simulink model "receiver_overall_reset"  (Simulink 7.5)
settings: Solver=FixedStepDiscrete  SolverMode=SingleTasking  StartTime=0.0  StopTime=(length(simin.signals.values)-1)/Fs  FixedStep=1  RelTol=1e-3
undefined symbols (not defined in the file): Fs
libraries: xbsIndex_r4 x962
(part 4 of 9)

== system receiver_overall_reset/Receiver/Sym-Chooser/6-14/Corr0 ==
  In1 : Inport
  AddSub : xbsIndex_r4/AddSub  mode=Subtraction  use_carryin=off  use_carryout=off  en=off  latency=0  precision=Full  arith_type=Unsigned  n_bits=16  bin_pt=14  quantization=Truncate  overflow=Wrap  dbl_ovrd=off  use_behavioral_HDL=off  hw_selection=Fabric  pipelined=off  block_type=addsub
      settings: xl_area=[4 0 0 6 0 0 0]  block_version=12.1
  Constant0 : xbsIndex_r4/Constant  arith_type=Unsigned  const=chip_a  n_bits=31  bin_pt=0  explicit_period=off  period=1/8  equ=P=C  opselect=C  inp2=PCIN>>17  opr=+  inp1=P  carry=CIN  dbl_ovrd=off  block_type=constant
      settings: block_version=12.1
  Constant1 : xbsIndex_r4/Constant  arith_type=Unsigned  const=31  n_bits=5  bin_pt=0  explicit_period=off  period=1/8  equ=P=C  opselect=C  inp2=PCIN>>17  opr=+  inp1=P  carry=CIN  dbl_ovrd=off  block_type=constant
      settings: block_version=12.1
  Corr : Subsystem
  Delay_Line : Subsystem  mask{bits=31}
      mask prompts: bits "Number of Bits [2-40]"
      mask init: same as receiver_overall_reset/Receiver/Sym-Clk/Corr/Delay_Line
      mask StyleString: popup(2|3|4|5|6|7|8|9|10|11|12|13|14|15|16|17|18|19|20|21|22|23|24|25|26|27|28|29|30|31|32|33|34|35|36|37|38|39|40)
  Logical : xbsIndex_r4/Logical  logical_function=XNOR  inputs=2  en=off  latency=0  precision=User Defined  arith_type=Unsigned  n_bits=32  bin_pt=0  align_bp=on  dbl_ovrd=off  block_type=logical
      settings: xl_area=[31 0 0 31 0 0 0]  block_version=12.1
  Shift : xbsIndex_r4/Shift  shift_dir=Left  shift_bits=1  en=off  latency=0  precision=Full  arith_type=Unsigned  n_bits=7  bin_pt=0  quantization=Truncate  overflow=Wrap  dbl_ovrd=off  block_type=shift
      settings: xl_area=[0 0 0 0 0 0 0]  block_version=12.1
  Out1 : Outport
  wires:
  Constant0/1 -> Logical/2
  Delay_Line/1(Out2) -> Logical/1
  Logical/1 -> Corr/1(In1)
  Constant1/1 -> AddSub/2
  Corr/1(Out2) -> Shift/1
  Shift/1 -> AddSub/1
  In1/1 -> Delay_Line/1(In1)
  AddSub/1 -> Out1/1

== system receiver_overall_reset/Receiver/Sym-Chooser/7-15/Corr0 ==
  In1 : Inport
  AddSub : xbsIndex_r4/AddSub  mode=Subtraction  use_carryin=off  use_carryout=off  en=off  latency=0  precision=Full  arith_type=Unsigned  n_bits=16  bin_pt=14  quantization=Truncate  overflow=Wrap  dbl_ovrd=off  use_behavioral_HDL=off  hw_selection=Fabric  pipelined=off  block_type=addsub
      settings: xl_area=[4 0 0 6 0 0 0]  block_version=12.1
  Constant0 : xbsIndex_r4/Constant  arith_type=Unsigned  const=chip_a  n_bits=31  bin_pt=0  explicit_period=off  period=1/8  equ=P=C  opselect=C  inp2=PCIN>>17  opr=+  inp1=P  carry=CIN  dbl_ovrd=off  block_type=constant
      settings: block_version=12.1
  Constant1 : xbsIndex_r4/Constant  arith_type=Unsigned  const=31  n_bits=5  bin_pt=0  explicit_period=off  period=1/8  equ=P=C  opselect=C  inp2=PCIN>>17  opr=+  inp1=P  carry=CIN  dbl_ovrd=off  block_type=constant
      settings: block_version=12.1
  Corr : Subsystem
  Delay_Line : Subsystem  mask{bits=31}
      mask prompts: bits "Number of Bits [2-40]"
      mask init: same as receiver_overall_reset/Receiver/Sym-Clk/Corr/Delay_Line
      mask StyleString: popup(2|3|4|5|6|7|8|9|10|11|12|13|14|15|16|17|18|19|20|21|22|23|24|25|26|27|28|29|30|31|32|33|34|35|36|37|38|39|40)
  Logical : xbsIndex_r4/Logical  logical_function=XNOR  inputs=2  en=off  latency=0  precision=User Defined  arith_type=Unsigned  n_bits=32  bin_pt=0  align_bp=on  dbl_ovrd=off  block_type=logical
      settings: xl_area=[31 0 0 31 0 0 0]  block_version=12.1
  Shift : xbsIndex_r4/Shift  shift_dir=Left  shift_bits=1  en=off  latency=0  precision=Full  arith_type=Unsigned  n_bits=7  bin_pt=0  quantization=Truncate  overflow=Wrap  dbl_ovrd=off  block_type=shift
      settings: xl_area=[0 0 0 0 0 0 0]  block_version=12.1
  Out1 : Outport
  wires:
  Constant0/1 -> Logical/2
  Delay_Line/1(Out2) -> Logical/1
  Logical/1 -> Corr/1(In1)
  Constant1/1 -> AddSub/2
  Corr/1(Out2) -> Shift/1
  Shift/1 -> AddSub/1
  In1/1 -> Delay_Line/1(In1)
  AddSub/1 -> Out1/1

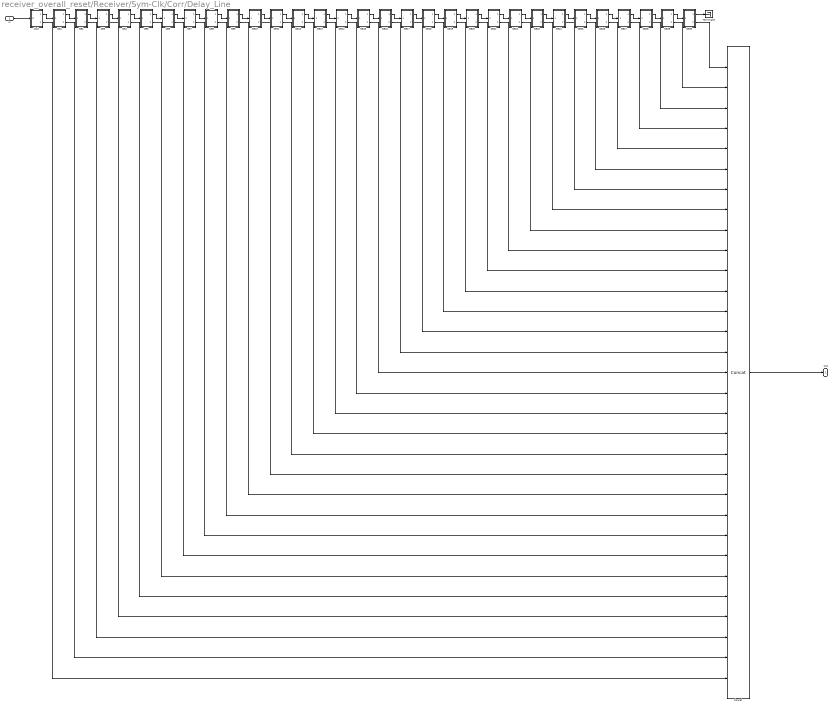
== system receiver_overall_reset/Receiver/Sym-Clk/Corr/Delay_Line ==
  In : Inport
  1to2 : Subsystem
  Concat : xbsIndex_r4/Concat  num_inputs=31  dbl_ovrd=off  block_type=concat
      settings: block_version=12.1
  DE1 : Subsystem
      mask Display: disp('z^{-1}','texmode','on')
  DE10 : Subsystem
      mask Display: disp('z^{-1}','texmode','on')
  DE11 : Subsystem
      mask Display: disp('z^{-1}','texmode','on')
  DE12 : Subsystem
      mask Display: disp('z^{-1}','texmode','on')
  DE13 : Subsystem
      mask Display: disp('z^{-1}','texmode','on')
  DE14 : Subsystem
      mask Display: disp('z^{-1}','texmode','on')
  DE15 : Subsystem
      mask Display: disp('z^{-1}','texmode','on')
  DE16 : Subsystem
      mask Display: disp('z^{-1}','texmode','on')
  DE17 : Subsystem
      mask Display: disp('z^{-1}','texmode','on')
  DE18 : Subsystem
      mask Display: disp('z^{-1}','texmode','on')
  DE19 : Subsystem
      mask Display: disp('z^{-1}','texmode','on')
  DE2 : Subsystem
      mask Display: disp('z^{-1}','texmode','on')
  DE20 : Subsystem
      mask Display: disp('z^{-1}','texmode','on')
  DE21 : Subsystem
      mask Display: disp('z^{-1}','texmode','on')
  DE22 : Subsystem
      mask Display: disp('z^{-1}','texmode','on')
  DE23 : Subsystem
      mask Display: disp('z^{-1}','texmode','on')
  DE24 : Subsystem
      mask Display: disp('z^{-1}','texmode','on')
  DE25 : Subsystem
      mask Display: disp('z^{-1}','texmode','on')
  DE26 : Subsystem
      mask Display: disp('z^{-1}','texmode','on')
  DE27 : Subsystem
      mask Display: disp('z^{-1}','texmode','on')
  DE28 : Subsystem
      mask Display: disp('z^{-1}','texmode','on')
  DE29 : Subsystem
      mask Display: disp('z^{-1}','texmode','on')
  DE3 : Subsystem
      mask Display: disp('z^{-1}','texmode','on')
  DE30 : Subsystem
      mask Display: disp('z^{-1}','texmode','on')
  DE4 : Subsystem
      mask Display: disp('z^{-1}','texmode','on')
  DE5 : Subsystem
      mask Display: disp('z^{-1}','texmode','on')
  DE6 : Subsystem
      mask Display: disp('z^{-1}','texmode','on')
  DE7 : Subsystem
      mask Display: disp('z^{-1}','texmode','on')
  DE8 : Subsystem
      mask Display: disp('z^{-1}','texmode','on')
  DE9 : Subsystem
      mask Display: disp('z^{-1}','texmode','on')
  Terminator : Terminator
  Out : Outport
  wires:
  Concat/1 -> Out/1
  In/1 -> 1to2/1(In)
  1to2/1(Out1) -> DE1/1(In1)
  DE30/1(Out1) -> Terminator/1
  1to2/2(Out2) -> Concat/31
  DE1/2(Out2) -> Concat/30
  DE2/2(Out2) -> Concat/29
  DE3/2(Out2) -> Concat/28
  DE4/2(Out2) -> Concat/27
  DE5/2(Out2) -> Concat/26
  DE6/2(Out2) -> Concat/25
  DE7/2(Out2) -> Concat/24
  DE8/2(Out2) -> Concat/23
  DE9/2(Out2) -> Concat/22
  DE10/2(Out2) -> Concat/21
  DE11/2(Out2) -> Concat/20
  DE12/2(Out2) -> Concat/19
  DE13/2(Out2) -> Concat/18
  DE14/2(Out2) -> Concat/17
  DE15/2(Out2) -> Concat/16
  DE16/2(Out2) -> Concat/15
  DE17/2(Out2) -> Concat/14
  DE18/2(Out2) -> Concat/13
  DE19/2(Out2) -> Concat/12
  DE20/2(Out2) -> Concat/11
  DE21/2(Out2) -> Concat/10
  DE22/2(Out2) -> Concat/9
  DE23/2(Out2) -> Concat/8
  DE24/2(Out2) -> Concat/7
  DE25/2(Out2) -> Concat/6
  DE26/2(Out2) -> Concat/5
  DE27/2(Out2) -> Concat/4
  DE28/2(Out2) -> Concat/3
  DE29/2(Out2) -> Concat/2
  DE30/2(Out2) -> Concat/1
  DE2/1(Out1) -> DE3/1(In1)
  DE3/1(Out1) -> DE4/1(In1)
  DE4/1(Out1) -> DE5/1(In1)
  DE5/1(Out1) -> DE6/1(In1)
  DE6/1(Out1) -> DE7/1(In1)
  DE7/1(Out1) -> DE8/1(In1)
  DE8/1(Out1) -> DE9/1(In1)
  DE9/1(Out1) -> DE10/1(In1)
  DE10/1(Out1) -> DE11/1(In1)
  DE11/1(Out1) -> DE12/1(In1)
  DE12/1(Out1) -> DE13/1(In1)
  DE13/1(Out1) -> DE14/1(In1)
  DE14/1(Out1) -> DE15/1(In1)
  DE15/1(Out1) -> DE16/1(In1)
  DE16/1(Out1) -> DE17/1(In1)
  DE17/1(Out1) -> DE18/1(In1)
  DE18/1(Out1) -> DE19/1(In1)
  DE19/1(Out1) -> DE20/1(In1)
  DE20/1(Out1) -> DE21/1(In1)
  DE21/1(Out1) -> DE22/1(In1)
  DE22/1(Out1) -> DE23/1(In1)
  DE23/1(Out1) -> DE24/1(In1)
  DE24/1(Out1) -> DE25/1(In1)
  DE25/1(Out1) -> DE26/1(In1)
  DE26/1(Out1) -> DE27/1(In1)
  DE27/1(Out1) -> DE28/1(In1)
  DE28/1(Out1) -> DE29/1(In1)
  DE29/1(Out1) -> DE30/1(In1)
  DE1/1(Out1) -> DE2/1(In1)

== system receiver_overall_reset/Receiver/Sym-Clk/Corr/count 1s ==
  in : Inport
  0-3 : xbsIndex_r4/Slice  nbits=4  boolean_output=off  mode=Lower Bit Location + Width  bit1=0  base1=MSB of Input  bit0=0  base0=LSB of Input  dbl_ovrd=off  block_type=slice
      settings: block_version=12.1
  12-15 : xbsIndex_r4/Slice  nbits=4  boolean_output=off  mode=Lower Bit Location + Width  bit1=-12  base1=MSB of Input  bit0=12  base0=LSB of Input  dbl_ovrd=off  block_type=slice
      settings: block_version=12.1
  16-19 : xbsIndex_r4/Slice  nbits=4  boolean_output=off  mode=Lower Bit Location + Width  bit1=0  base1=LSB of Input  bit0=16  base0=LSB of Input  dbl_ovrd=off  block_type=slice
      settings: block_version=12.1
  20-23 : xbsIndex_r4/Slice  nbits=4  boolean_output=off  mode=Lower Bit Location + Width  bit1=0  base1=LSB of Input  bit0=20  base0=LSB of Input  dbl_ovrd=off  block_type=slice
      settings: block_version=12.1
  24-27 : xbsIndex_r4/Slice  nbits=4  boolean_output=off  mode=Lower Bit Location + Width  bit1=0  base1=LSB of Input  bit0=24  base0=LSB of Input  dbl_ovrd=off  block_type=slice
      settings: block_version=12.1
  28-31 : xbsIndex_r4/Slice  nbits=4  boolean_output=off  mode=Lower Bit Location + Width  bit1=0  base1=LSB of Input  bit0=28  base0=LSB of Input  dbl_ovrd=off  block_type=slice
      settings: block_version=12.1
  4-7 : xbsIndex_r4/Slice  nbits=4  boolean_output=off  mode=Lower Bit Location + Width  bit1=-4  base1=MSB of Input  bit0=4  base0=LSB of Input  dbl_ovrd=off  block_type=slice
      settings: block_version=12.1
  8-11 : xbsIndex_r4/Slice  nbits=4  boolean_output=off  mode=Lower Bit Location + Width  bit1=-8  base1=MSB of Input  bit0=8  base0=LSB of Input  dbl_ovrd=off  block_type=slice
      settings: block_version=12.1
  AddSub2 : xbsIndex_r4/AddSub  mode=Addition  use_carryin=off  use_carryout=off  en=off  latency=0  precision=Full  arith_type=Unsigned  n_bits=16  bin_pt=14  quantization=Truncate  overflow=Wrap  dbl_ovrd=off  use_behavioral_HDL=off  hw_selection=Fabric  pipelined=off  block_type=addsub
      settings: xl_area=[3 0 0 4 0 0 0]  block_version=12.1
  AddSub3 : xbsIndex_r4/AddSub  mode=Addition  use_carryin=off  use_carryout=off  en=off  latency=0  precision=Full  arith_type=Unsigned  n_bits=16  bin_pt=14  quantization=Truncate  overflow=Wrap  dbl_ovrd=off  use_behavioral_HDL=off  hw_selection=Fabric  pipelined=off  block_type=addsub
      settings: xl_area=[3 0 0 5 0 0 0]  block_version=12.1
  AddSub6 : xbsIndex_r4/AddSub  mode=Addition  use_carryin=off  use_carryout=off  en=off  latency=0  precision=Full  arith_type=Unsigned  n_bits=16  bin_pt=14  quantization=Truncate  overflow=Wrap  dbl_ovrd=off  use_behavioral_HDL=off  hw_selection=Fabric  pipelined=off  block_type=addsub
      settings: xl_area=[3 0 0 4 0 0 0]  block_version=12.1
  LUT{0..7} (8 alike) : xbsIndex_r4/ROM  depth=16  initVector=[0,1,1,2,1,2,2,3,1,2,2,3,2,3,3,4]  distributed_mem=Distributed memory  rst=off  init_reg=0  en=off  latency=0  arith_type=Unsigned  n_bits=3  bin_pt=0  dbl_ovrd=off  optimize=Area  use_rpm=on  block_type=sprom
      settings: xl_area=[0 0 1 0 0 0 0]  block_version=12.1
  add{1..4} (4 alike) : xbsIndex_r4/AddSub  mode=Addition  use_carryin=off  use_carryout=off  en=off  latency=0  precision=Full  arith_type=Unsigned  n_bits=16  bin_pt=14  quantization=Truncate  overflow=Wrap  dbl_ovrd=off  use_behavioral_HDL=off  hw_selection=Fabric  pipelined=off  block_type=addsub
      settings: xl_area=[2 0 0 3 0 0 0]  block_version=12.1
  out : Outport
  wires:
  in/1 -> 0-3/1, 12-15/1, 28-31/1, 24-27/1, 20-23/1, 16-19/1, 8-11/1, 4-7/1
  0-3/1 -> LUT0/1
  12-15/1 -> LUT3/1
  8-11/1 -> LUT2/1
  4-7/1 -> LUT1/1
  LUT0/1 -> add1/1
  LUT1/1 -> add1/2
  LUT2/1 -> add2/1
  LUT3/1 -> add2/2
  add2/1 -> AddSub2/2
  add1/1 -> AddSub2/1
  AddSub3/1 -> out/1
  16-19/1 -> LUT4/1
  28-31/1 -> LUT7/1
  24-27/1 -> LUT6/1
  20-23/1 -> LUT5/1
  LUT4/1 -> add3/1
  LUT5/1 -> add3/2
  LUT6/1 -> add4/1
  LUT7/1 -> add4/2
  add4/1 -> AddSub6/2
  add3/1 -> AddSub6/1
  AddSub2/1 -> AddSub3/1
  AddSub6/1 -> AddSub3/2

== system receiver_overall_reset/Receiver/FM demod/CORDIC ATAN/CORDIC Fine Angle PE/CORDIC PE1 ==
  note: X = x - y if y < 0, otherwise
      |    = x + y
      | Y = y + x if y < 0, otherwise
      |    = y - x
      | Z = z - atan(1/2^i) if y < 0, otherwise
      |    = z + atan(1/2^i)
  x : Inport  OutDataType=sfix(16)  OutScaling=2^0
  y : Inport  Port=2  OutDataType=sfix(16)  OutScaling=2^0
  z : Inport  Port=3  OutDataType=sfix(16)  OutScaling=2^0
  AddSub : xbsIndex_r4/AddSub  mode=Addition or Subtraction  use_carryin=off  use_carryout=off  en=off  latency=pipeline  precision=User Defined  arith_type="Signed  (2's comp)"  n_bits=pe_nbits  bin_pt=pe_binpt  quantization=Truncate  overflow=Wrap  dbl_ovrd=off  use_behavioral_HDL=on  hw_selection=Fabric  pipelined=off  use_rpm=off  block_type=addsub
      settings: xl_area=[17 0 0 33 0 0 0]  block_version=VER_STRING_GOES_HERE
  AddSub1 : xbsIndex_r4/AddSub  mode=Addition or Subtraction  use_carryin=off  use_carryout=off  en=off  latency=pipeline  precision=User Defined  arith_type="Signed  (2's comp)"  n_bits=pe_nbits  bin_pt=pe_binpt  quantization=Truncate  overflow=Wrap  dbl_ovrd=off  use_behavioral_HDL=on  hw_selection=Fabric  pipelined=off  use_rpm=off  block_type=addsub
      settings: xl_area=[17 0 0 33 0 0 0]  block_version=VER_STRING_GOES_HERE
  AddSub2 : xbsIndex_r4/AddSub  mode=Addition or Subtraction  use_carryin=off  use_carryout=off  en=off  latency=pipeline  precision=User Defined  arith_type="Signed  (2's comp)"  n_bits=pe_nbits  bin_pt=pe_binpt  quantization=Truncate  overflow=Wrap  dbl_ovrd=off  use_behavioral_HDL=on  hw_selection=Fabric  pipelined=off  use_rpm=off  block_type=addsub
      settings: xl_area=[17 0 0 33 0 0 0]  block_version=VER_STRING_GOES_HERE
  Constant : xbsIndex_r4/Constant  arith_type=Signed (2's comp)  const=epsilon_k  n_bits=pe_nbits  bin_pt=pe_binpt  explicit_period=off  period=1  equ=P=C  opselect=C  inp2=PCIN>>17  opr=+  inp1=P  carry=CIN  dbl_ovrd=off  block_type=constant
      settings: block_version=VER_STRING_GOES_HERE
  Inverter : xbsIndex_r4/Inverter  en=off  latency=0  dbl_ovrd=off  block_type=inv
      settings: xl_area=[0 0 0 0 0 0 0]  block_version=VER_STRING_GOES_HERE
  Shift : xbsIndex_r4/Shift  shift_dir=Right  shift_bits=ii  en=off  latency=0  precision=User Defined  arith_type="Signed  (2's comp)"  n_bits=pe_nbits  bin_pt=pe_binpt  quantization=Truncate  overflow=Wrap  dbl_ovrd=off  block_type=shift
      settings: xl_area=[0 0 0 0 0 0 0]  block_version=VER_STRING_GOES_HERE
  Shift1 : xbsIndex_r4/Shift  shift_dir=Right  shift_bits=ii  en=off  latency=0  precision=User Defined  arith_type="Signed  (2's comp)"  n_bits=pe_nbits  bin_pt=pe_binpt  quantization=Truncate  overflow=Wrap  dbl_ovrd=off  block_type=shift
      settings: xl_area=[0 0 0 0 0 0 0]  block_version=VER_STRING_GOES_HERE
  Slice : xbsIndex_r4/Slice  nbits=1  boolean_output=on  mode=Upper Bit Location + Width  bit1=0  base1=MSB of Input  bit0=0  base0=LSB of Input  dbl_ovrd=off  block_type=slice
      settings: infoedit="Extracts a given range of bits from each input sample and presents it at the output.  The output type is ordinarily unsigned with binary point at zero, but can be Boolean when the slice is one bit wide.<P><P>Hardware notes: In hardware this block costs nothing."  block_version=VER_STRING_GOES_HERE
  X : Outport  OutDataType=sfix(16)  OutScaling=2^0
  Y : Outport  Port=2  OutDataType=sfix(16)  OutScaling=2^0
  Z : Outport  Port=3  OutDataType=sfix(16)  OutScaling=2^0
  wires:
  Slice/1 -> AddSub/3, AddSub2/3, Inverter/1
  Shift1/1 -> AddSub/2
  Shift/1 -> AddSub1/2
  Inverter/1 -> AddSub1/3
  Constant/1 -> AddSub2/2
  AddSub2/1 -> Z/1
  AddSub1/1 -> Y/1
  z/1 -> AddSub2/1
  AddSub/1 -> X/1
  y/1 -> Slice/1, Shift1/1, AddSub1/1
  x/1 -> Shift/1, AddSub/1

== system receiver_overall_reset/Receiver/FM demod/CORDIC ATAN/CORDIC Fine Angle PE/CORDIC PE2 ==
  note: X = x - y if y < 0, otherwise
      |    = x + y
      | Y = y + x if y < 0, otherwise
      |    = y - x
      | Z = z - atan(1/2^i) if y < 0, otherwise
      |    = z + atan(1/2^i)
  x : Inport  OutDataType=sfix(16)  OutScaling=2^0
  y : Inport  Port=2  OutDataType=sfix(16)  OutScaling=2^0
  z : Inport  Port=3  OutDataType=sfix(16)  OutScaling=2^0
  AddSub : xbsIndex_r4/AddSub  mode=Addition or Subtraction  use_carryin=off  use_carryout=off  en=off  latency=pipeline  precision=User Defined  arith_type="Signed  (2's comp)"  n_bits=pe_nbits  bin_pt=pe_binpt  quantization=Truncate  overflow=Wrap  dbl_ovrd=off  use_behavioral_HDL=on  hw_selection=Fabric  pipelined=off  use_rpm=off  block_type=addsub
      settings: xl_area=[17 0 0 33 0 0 0]  block_version=VER_STRING_GOES_HERE
  AddSub1 : xbsIndex_r4/AddSub  mode=Addition or Subtraction  use_carryin=off  use_carryout=off  en=off  latency=pipeline  precision=User Defined  arith_type="Signed  (2's comp)"  n_bits=pe_nbits  bin_pt=pe_binpt  quantization=Truncate  overflow=Wrap  dbl_ovrd=off  use_behavioral_HDL=on  hw_selection=Fabric  pipelined=off  use_rpm=off  block_type=addsub
      settings: xl_area=[17 0 0 33 0 0 0]  block_version=VER_STRING_GOES_HERE
  AddSub2 : xbsIndex_r4/AddSub  mode=Addition or Subtraction  use_carryin=off  use_carryout=off  en=off  latency=pipeline  precision=User Defined  arith_type="Signed  (2's comp)"  n_bits=pe_nbits  bin_pt=pe_binpt  quantization=Truncate  overflow=Wrap  dbl_ovrd=off  use_behavioral_HDL=on  hw_selection=Fabric  pipelined=off  use_rpm=off  block_type=addsub
      settings: xl_area=[17 0 0 33 0 0 0]  block_version=VER_STRING_GOES_HERE
  Constant : xbsIndex_r4/Constant  arith_type=Signed (2's comp)  const=epsilon_k  n_bits=pe_nbits  bin_pt=pe_binpt  explicit_period=off  period=1  equ=P=C  opselect=C  inp2=PCIN>>17  opr=+  inp1=P  carry=CIN  dbl_ovrd=off  block_type=constant
      settings: block_version=VER_STRING_GOES_HERE
  Inverter : xbsIndex_r4/Inverter  en=off  latency=0  dbl_ovrd=off  block_type=inv
      settings: xl_area=[0 0 0 0 0 0 0]  block_version=VER_STRING_GOES_HERE
  Shift : xbsIndex_r4/Shift  shift_dir=Right  shift_bits=ii  en=off  latency=0  precision=User Defined  arith_type="Signed  (2's comp)"  n_bits=pe_nbits  bin_pt=pe_binpt  quantization=Truncate  overflow=Wrap  dbl_ovrd=off  block_type=shift
      settings: xl_area=[0 0 0 0 0 0 0]  block_version=VER_STRING_GOES_HERE
  Shift1 : xbsIndex_r4/Shift  shift_dir=Right  shift_bits=ii  en=off  latency=0  precision=User Defined  arith_type="Signed  (2's comp)"  n_bits=pe_nbits  bin_pt=pe_binpt  quantization=Truncate  overflow=Wrap  dbl_ovrd=off  block_type=shift
      settings: xl_area=[0 0 0 0 0 0 0]  block_version=VER_STRING_GOES_HERE
  Slice : xbsIndex_r4/Slice  nbits=1  boolean_output=on  mode=Upper Bit Location + Width  bit1=0  base1=MSB of Input  bit0=0  base0=LSB of Input  dbl_ovrd=off  block_type=slice
      settings: infoedit="Extracts a given range of bits from each input sample and presents it at the output.  The output type is ordinarily unsigned with binary point at zero, but can be Boolean when the slice is one bit wide.<P><P>Hardware notes: In hardware this block costs nothing."  block_version=VER_STRING_GOES_HERE
  X : Outport  OutDataType=sfix(16)  OutScaling=2^0
  Y : Outport  Port=2  OutDataType=sfix(16)  OutScaling=2^0
  Z : Outport  Port=3  OutDataType=sfix(16)  OutScaling=2^0
  wires:
  x/1 -> AddSub/1, Shift/1
  y/1 -> AddSub1/1, Shift1/1, Slice/1
  AddSub/1 -> X/1
  z/1 -> AddSub2/1
  AddSub1/1 -> Y/1
  AddSub2/1 -> Z/1
  Constant/1 -> AddSub2/2
  Inverter/1 -> AddSub1/3
  Shift/1 -> AddSub1/2
  Shift1/1 -> AddSub/2
  Slice/1 -> Inverter/1, AddSub2/3, AddSub/3

== system receiver_overall_reset/Receiver/FM demod/CORDIC ATAN/CORDIC Fine Angle PE/CORDIC PE3 ==
  note: X = x - y if y < 0, otherwise
      |    = x + y
      | Y = y + x if y < 0, otherwise
      |    = y - x
      | Z = z - atan(1/2^i) if y < 0, otherwise
      |    = z + atan(1/2^i)
  x : Inport  OutDataType=sfix(16)  OutScaling=2^0
  y : Inport  Port=2  OutDataType=sfix(16)  OutScaling=2^0
  z : Inport  Port=3  OutDataType=sfix(16)  OutScaling=2^0
  AddSub : xbsIndex_r4/AddSub  mode=Addition or Subtraction  use_carryin=off  use_carryout=off  en=off  latency=pipeline  precision=User Defined  arith_type="Signed  (2's comp)"  n_bits=pe_nbits  bin_pt=pe_binpt  quantization=Truncate  overflow=Wrap  dbl_ovrd=off  use_behavioral_HDL=on  hw_selection=Fabric  pipelined=off  use_rpm=off  block_type=addsub
      settings: xl_area=[17 0 0 33 0 0 0]  block_version=VER_STRING_GOES_HERE
  AddSub1 : xbsIndex_r4/AddSub  mode=Addition or Subtraction  use_carryin=off  use_carryout=off  en=off  latency=pipeline  precision=User Defined  arith_type="Signed  (2's comp)"  n_bits=pe_nbits  bin_pt=pe_binpt  quantization=Truncate  overflow=Wrap  dbl_ovrd=off  use_behavioral_HDL=on  hw_selection=Fabric  pipelined=off  use_rpm=off  block_type=addsub
      settings: xl_area=[17 0 0 33 0 0 0]  block_version=VER_STRING_GOES_HERE
  AddSub2 : xbsIndex_r4/AddSub  mode=Addition or Subtraction  use_carryin=off  use_carryout=off  en=off  latency=pipeline  precision=User Defined  arith_type="Signed  (2's comp)"  n_bits=pe_nbits  bin_pt=pe_binpt  quantization=Truncate  overflow=Wrap  dbl_ovrd=off  use_behavioral_HDL=on  hw_selection=Fabric  pipelined=off  use_rpm=off  block_type=addsub
      settings: xl_area=[17 0 0 33 0 0 0]  block_version=VER_STRING_GOES_HERE
  Constant : xbsIndex_r4/Constant  arith_type=Signed (2's comp)  const=epsilon_k  n_bits=pe_nbits  bin_pt=pe_binpt  explicit_period=off  period=1  equ=P=C  opselect=C  inp2=PCIN>>17  opr=+  inp1=P  carry=CIN  dbl_ovrd=off  block_type=constant
      settings: block_version=VER_STRING_GOES_HERE
  Inverter : xbsIndex_r4/Inverter  en=off  latency=0  dbl_ovrd=off  block_type=inv
      settings: xl_area=[0 0 0 0 0 0 0]  block_version=VER_STRING_GOES_HERE
  Shift : xbsIndex_r4/Shift  shift_dir=Right  shift_bits=ii  en=off  latency=0  precision=User Defined  arith_type="Signed  (2's comp)"  n_bits=pe_nbits  bin_pt=pe_binpt  quantization=Truncate  overflow=Wrap  dbl_ovrd=off  block_type=shift
      settings: xl_area=[0 0 0 0 0 0 0]  block_version=VER_STRING_GOES_HERE
  Shift1 : xbsIndex_r4/Shift  shift_dir=Right  shift_bits=ii  en=off  latency=0  precision=User Defined  arith_type="Signed  (2's comp)"  n_bits=pe_nbits  bin_pt=pe_binpt  quantization=Truncate  overflow=Wrap  dbl_ovrd=off  block_type=shift
      settings: xl_area=[0 0 0 0 0 0 0]  block_version=VER_STRING_GOES_HERE
  Slice : xbsIndex_r4/Slice  nbits=1  boolean_output=on  mode=Upper Bit Location + Width  bit1=0  base1=MSB of Input  bit0=0  base0=LSB of Input  dbl_ovrd=off  block_type=slice
      settings: infoedit="Extracts a given range of bits from each input sample and presents it at the output.  The output type is ordinarily unsigned with binary point at zero, but can be Boolean when the slice is one bit wide.<P><P>Hardware notes: In hardware this block costs nothing."  block_version=VER_STRING_GOES_HERE
  X : Outport  OutDataType=sfix(16)  OutScaling=2^0
  Y : Outport  Port=2  OutDataType=sfix(16)  OutScaling=2^0
  Z : Outport  Port=3  OutDataType=sfix(16)  OutScaling=2^0
  wires:
  x/1 -> AddSub/1, Shift/1
  y/1 -> AddSub1/1, Shift1/1, Slice/1
  AddSub/1 -> X/1
  z/1 -> AddSub2/1
  AddSub1/1 -> Y/1
  AddSub2/1 -> Z/1
  Constant/1 -> AddSub2/2
  Inverter/1 -> AddSub1/3
  Shift/1 -> AddSub1/2
  Shift1/1 -> AddSub/2
  Slice/1 -> Inverter/1, AddSub2/3, AddSub/3

== system receiver_overall_reset/Receiver/FM demod/CORDIC ATAN/CORDIC Fine Angle PE/CORDIC PE4 ==
  note: X = x - y if y < 0, otherwise
      |    = x + y
      | Y = y + x if y < 0, otherwise
      |    = y - x
      | Z = z - atan(1/2^i) if y < 0, otherwise
      |    = z + atan(1/2^i)
  x : Inport  OutDataType=sfix(16)  OutScaling=2^0
  y : Inport  Port=2  OutDataType=sfix(16)  OutScaling=2^0
  z : Inport  Port=3  OutDataType=sfix(16)  OutScaling=2^0
  AddSub : xbsIndex_r4/AddSub  mode=Addition or Subtraction  use_carryin=off  use_carryout=off  en=off  latency=pipeline  precision=User Defined  arith_type="Signed  (2's comp)"  n_bits=pe_nbits  bin_pt=pe_binpt  quantization=Truncate  overflow=Wrap  dbl_ovrd=off  use_behavioral_HDL=on  hw_selection=Fabric  pipelined=off  use_rpm=off  block_type=addsub
      settings: xl_area=[17 0 0 33 0 0 0]  block_version=VER_STRING_GOES_HERE
  AddSub1 : xbsIndex_r4/AddSub  mode=Addition or Subtraction  use_carryin=off  use_carryout=off  en=off  latency=pipeline  precision=User Defined  arith_type="Signed  (2's comp)"  n_bits=pe_nbits  bin_pt=pe_binpt  quantization=Truncate  overflow=Wrap  dbl_ovrd=off  use_behavioral_HDL=on  hw_selection=Fabric  pipelined=off  use_rpm=off  block_type=addsub
      settings: xl_area=[17 0 0 33 0 0 0]  block_version=VER_STRING_GOES_HERE
  AddSub2 : xbsIndex_r4/AddSub  mode=Addition or Subtraction  use_carryin=off  use_carryout=off  en=off  latency=pipeline  precision=User Defined  arith_type="Signed  (2's comp)"  n_bits=pe_nbits  bin_pt=pe_binpt  quantization=Truncate  overflow=Wrap  dbl_ovrd=off  use_behavioral_HDL=on  hw_selection=Fabric  pipelined=off  use_rpm=off  block_type=addsub
      settings: xl_area=[17 0 0 33 0 0 0]  block_version=VER_STRING_GOES_HERE
  Constant : xbsIndex_r4/Constant  arith_type=Signed (2's comp)  const=epsilon_k  n_bits=pe_nbits  bin_pt=pe_binpt  explicit_period=off  period=1  equ=P=C  opselect=C  inp2=PCIN>>17  opr=+  inp1=P  carry=CIN  dbl_ovrd=off  block_type=constant
      settings: block_version=VER_STRING_GOES_HERE
  Inverter : xbsIndex_r4/Inverter  en=off  latency=0  dbl_ovrd=off  block_type=inv
      settings: xl_area=[0 0 0 0 0 0 0]  block_version=VER_STRING_GOES_HERE
  Shift : xbsIndex_r4/Shift  shift_dir=Right  shift_bits=ii  en=off  latency=0  precision=User Defined  arith_type="Signed  (2's comp)"  n_bits=pe_nbits  bin_pt=pe_binpt  quantization=Truncate  overflow=Wrap  dbl_ovrd=off  block_type=shift
      settings: xl_area=[0 0 0 0 0 0 0]  block_version=VER_STRING_GOES_HERE
  Shift1 : xbsIndex_r4/Shift  shift_dir=Right  shift_bits=ii  en=off  latency=0  precision=User Defined  arith_type="Signed  (2's comp)"  n_bits=pe_nbits  bin_pt=pe_binpt  quantization=Truncate  overflow=Wrap  dbl_ovrd=off  block_type=shift
      settings: xl_area=[0 0 0 0 0 0 0]  block_version=VER_STRING_GOES_HERE
  Slice : xbsIndex_r4/Slice  nbits=1  boolean_output=on  mode=Upper Bit Location + Width  bit1=0  base1=MSB of Input  bit0=0  base0=LSB of Input  dbl_ovrd=off  block_type=slice
      settings: infoedit="Extracts a given range of bits from each input sample and presents it at the output.  The output type is ordinarily unsigned with binary point at zero, but can be Boolean when the slice is one bit wide.<P><P>Hardware notes: In hardware this block costs nothing."  block_version=VER_STRING_GOES_HERE
  X : Outport  OutDataType=sfix(16)  OutScaling=2^0
  Y : Outport  Port=2  OutDataType=sfix(16)  OutScaling=2^0
  Z : Outport  Port=3  OutDataType=sfix(16)  OutScaling=2^0
  wires:
  x/1 -> AddSub/1, Shift/1
  y/1 -> AddSub1/1, Shift1/1, Slice/1
  AddSub/1 -> X/1
  z/1 -> AddSub2/1
  AddSub1/1 -> Y/1
  AddSub2/1 -> Z/1
  Constant/1 -> AddSub2/2
  Inverter/1 -> AddSub1/3
  Shift/1 -> AddSub1/2
  Shift1/1 -> AddSub/2
  Slice/1 -> Inverter/1, AddSub2/3, AddSub/3

== system receiver_overall_reset/Receiver/FM demod/CORDIC ATAN/CORDIC Fine Angle PE/CORDIC PE5 ==
  note: X = x - y if y < 0, otherwise
      |    = x + y
      | Y = y + x if y < 0, otherwise
      |    = y - x
      | Z = z - atan(1/2^i) if y < 0, otherwise
      |    = z + atan(1/2^i)
  x : Inport  OutDataType=sfix(16)  OutScaling=2^0
  y : Inport  Port=2  OutDataType=sfix(16)  OutScaling=2^0
  z : Inport  Port=3  OutDataType=sfix(16)  OutScaling=2^0
  AddSub : xbsIndex_r4/AddSub  mode=Addition or Subtraction  use_carryin=off  use_carryout=off  en=off  latency=pipeline  precision=User Defined  arith_type="Signed  (2's comp)"  n_bits=pe_nbits  bin_pt=pe_binpt  quantization=Truncate  overflow=Wrap  dbl_ovrd=off  use_behavioral_HDL=on  hw_selection=Fabric  pipelined=off  use_rpm=off  block_type=addsub
      settings: xl_area=[17 0 0 33 0 0 0]  block_version=VER_STRING_GOES_HERE
  AddSub1 : xbsIndex_r4/AddSub  mode=Addition or Subtraction  use_carryin=off  use_carryout=off  en=off  latency=pipeline  precision=User Defined  arith_type="Signed  (2's comp)"  n_bits=pe_nbits  bin_pt=pe_binpt  quantization=Truncate  overflow=Wrap  dbl_ovrd=off  use_behavioral_HDL=on  hw_selection=Fabric  pipelined=off  use_rpm=off  block_type=addsub
      settings: xl_area=[17 0 0 33 0 0 0]  block_version=VER_STRING_GOES_HERE
  AddSub2 : xbsIndex_r4/AddSub  mode=Addition or Subtraction  use_carryin=off  use_carryout=off  en=off  latency=pipeline  precision=User Defined  arith_type="Signed  (2's comp)"  n_bits=pe_nbits  bin_pt=pe_binpt  quantization=Truncate  overflow=Wrap  dbl_ovrd=off  use_behavioral_HDL=on  hw_selection=Fabric  pipelined=off  use_rpm=off  block_type=addsub
      settings: xl_area=[17 0 0 33 0 0 0]  block_version=VER_STRING_GOES_HERE
  Constant : xbsIndex_r4/Constant  arith_type=Signed (2's comp)  const=epsilon_k  n_bits=pe_nbits  bin_pt=pe_binpt  explicit_period=off  period=1  equ=P=C  opselect=C  inp2=PCIN>>17  opr=+  inp1=P  carry=CIN  dbl_ovrd=off  block_type=constant
      settings: block_version=VER_STRING_GOES_HERE
  Inverter : xbsIndex_r4/Inverter  en=off  latency=0  dbl_ovrd=off  block_type=inv
      settings: xl_area=[0 0 0 0 0 0 0]  block_version=VER_STRING_GOES_HERE
  Shift : xbsIndex_r4/Shift  shift_dir=Right  shift_bits=ii  en=off  latency=0  precision=User Defined  arith_type="Signed  (2's comp)"  n_bits=pe_nbits  bin_pt=pe_binpt  quantization=Truncate  overflow=Wrap  dbl_ovrd=off  block_type=shift
      settings: xl_area=[0 0 0 0 0 0 0]  block_version=VER_STRING_GOES_HERE
  Shift1 : xbsIndex_r4/Shift  shift_dir=Right  shift_bits=ii  en=off  latency=0  precision=User Defined  arith_type="Signed  (2's comp)"  n_bits=pe_nbits  bin_pt=pe_binpt  quantization=Truncate  overflow=Wrap  dbl_ovrd=off  block_type=shift
      settings: xl_area=[0 0 0 0 0 0 0]  block_version=VER_STRING_GOES_HERE
  Slice : xbsIndex_r4/Slice  nbits=1  boolean_output=on  mode=Upper Bit Location + Width  bit1=0  base1=MSB of Input  bit0=0  base0=LSB of Input  dbl_ovrd=off  block_type=slice
      settings: infoedit="Extracts a given range of bits from each input sample and presents it at the output.  The output type is ordinarily unsigned with binary point at zero, but can be Boolean when the slice is one bit wide.<P><P>Hardware notes: In hardware this block costs nothing."  block_version=VER_STRING_GOES_HERE
  X : Outport  OutDataType=sfix(16)  OutScaling=2^0
  Y : Outport  Port=2  OutDataType=sfix(16)  OutScaling=2^0
  Z : Outport  Port=3  OutDataType=sfix(16)  OutScaling=2^0
  wires:
  x/1 -> AddSub/1, Shift/1
  y/1 -> AddSub1/1, Shift1/1, Slice/1
  AddSub/1 -> X/1
  z/1 -> AddSub2/1
  AddSub1/1 -> Y/1
  AddSub2/1 -> Z/1
  Constant/1 -> AddSub2/2
  Inverter/1 -> AddSub1/3
  Shift/1 -> AddSub1/2
  Shift1/1 -> AddSub/2
  Slice/1 -> Inverter/1, AddSub2/3, AddSub/3

== system receiver_overall_reset/Receiver/Sym-Chooser/0-8/Corr0/Corr ==
  In1 : Inport
  AddSub{,1..6} (7 alike) : xbsIndex_r4/AddSub  mode=Addition  use_carryin=off  use_carryout=off  en=off  latency=0  precision=Full  arith_type=Unsigned  n_bits=16  bin_pt=14  quantization=Truncate  overflow=Wrap  dbl_ovrd=off  use_behavioral_HDL=off  hw_selection=Fabric  pipelined=off  block_type=addsub
      AddSub settings: xl_area=[2 0 0 3 0 0 0]  block_version=12.1
      AddSub1 settings: xl_area=[2 0 0 3 0 0 0]  block_version=12.1
      AddSub2 settings: xl_area=[3 0 0 4 0 0 0]  block_version=12.1
      AddSub3 settings: xl_area=[3 0 0 5 0 0 0]  block_version=12.1
      AddSub4 settings: xl_area=[2 0 0 3 0 0 0]  block_version=12.1
      AddSub5 settings: xl_area=[2 0 0 3 0 0 0]  block_version=12.1
      AddSub6 settings: xl_area=[3 0 0 4 0 0 0]  block_version=12.1
  LUT{0..7} (8 alike) : xbsIndex_r4/ROM  depth=16  initVector=[0,1,1,2,1,2,2,3,1,2,2,3,2,3,3,4]  distributed_mem=Distributed memory  rst=off  init_reg=0  en=off  latency=0  arith_type=Unsigned  n_bits=3  bin_pt=0  dbl_ovrd=off  optimize=Area  use_rpm=on  block_type=sprom
      settings: xl_area=[0 0 1 0 0 0 0]  block_version=12.1
  Slice0 : xbsIndex_r4/Slice  nbits=4  boolean_output=off  mode=Lower Bit Location + Width  bit1=0  base1=MSB of Input  bit0=0  base0=LSB of Input  dbl_ovrd=off  block_type=slice
      settings: block_version=12.1
  Slice1 : xbsIndex_r4/Slice  nbits=4  boolean_output=off  mode=Lower Bit Location + Width  bit1=-4  base1=MSB of Input  bit0=4  base0=LSB of Input  dbl_ovrd=off  block_type=slice
      settings: block_version=12.1
  Slice2 : xbsIndex_r4/Slice  nbits=4  boolean_output=off  mode=Lower Bit Location + Width  bit1=-8  base1=MSB of Input  bit0=8  base0=LSB of Input  dbl_ovrd=off  block_type=slice
      settings: block_version=12.1
  Slice3 : xbsIndex_r4/Slice  nbits=4  boolean_output=off  mode=Lower Bit Location + Width  bit1=-12  base1=MSB of Input  bit0=12  base0=LSB of Input  dbl_ovrd=off  block_type=slice
      settings: block_version=12.1
  Slice4 : xbsIndex_r4/Slice  nbits=4  boolean_output=off  mode=Lower Bit Location + Width  bit1=0  base1=LSB of Input  bit0=16  base0=LSB of Input  dbl_ovrd=off  block_type=slice
      settings: block_version=12.1
  Slice5 : xbsIndex_r4/Slice  nbits=4  boolean_output=off  mode=Lower Bit Location + Width  bit1=0  base1=LSB of Input  bit0=20  base0=LSB of Input  dbl_ovrd=off  block_type=slice
      settings: block_version=12.1
  Slice6 : xbsIndex_r4/Slice  nbits=4  boolean_output=off  mode=Lower Bit Location + Width  bit1=0  base1=LSB of Input  bit0=24  base0=LSB of Input  dbl_ovrd=off  block_type=slice
      settings: block_version=12.1
  Slice7 : xbsIndex_r4/Slice  nbits=4  boolean_output=off  mode=Lower Bit Location + Width  bit1=0  base1=LSB of Input  bit0=28  base0=LSB of Input  dbl_ovrd=off  block_type=slice
      settings: block_version=12.1
  Out2 : Outport
  wires:
  In1/1 -> Slice0/1, Slice1/1, Slice2/1, Slice7/1, Slice6/1, Slice3/1, Slice4/1, Slice5/1
  Slice0/1 -> LUT0/1
  Slice3/1 -> LUT3/1
  Slice2/1 -> LUT2/1
  Slice1/1 -> LUT1/1
  LUT0/1 -> AddSub/1
  LUT1/1 -> AddSub/2
  LUT2/1 -> AddSub1/1
  LUT3/1 -> AddSub1/2
  AddSub1/1 -> AddSub2/2
  AddSub/1 -> AddSub2/1
  AddSub3/1 -> Out2/1
  Slice4/1 -> LUT4/1
  Slice7/1 -> LUT7/1
  Slice6/1 -> LUT6/1
  Slice5/1 -> LUT5/1
  LUT4/1 -> AddSub4/1
  LUT5/1 -> AddSub4/2
  LUT6/1 -> AddSub5/1
  LUT7/1 -> AddSub5/2
  AddSub5/1 -> AddSub6/2
  AddSub4/1 -> AddSub6/1
  AddSub2/1 -> AddSub3/1
  AddSub6/1 -> AddSub3/2

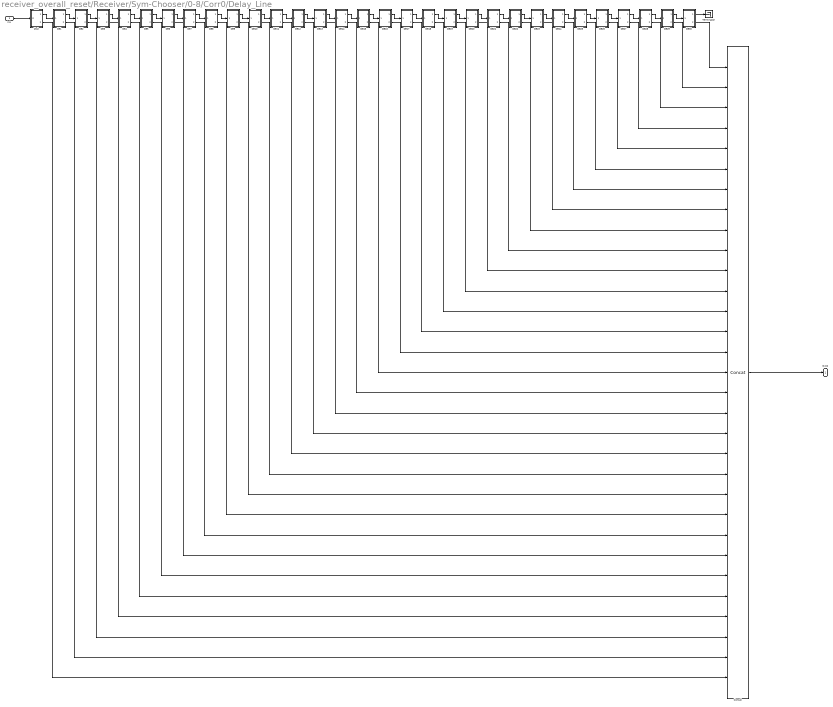
== system receiver_overall_reset/Receiver/Sym-Chooser/0-8/Corr0/Delay_Line ==
  In1 : Inport
  1to2 : Subsystem
  Concat : xbsIndex_r4/Concat  num_inputs=31  dbl_ovrd=off  block_type=concat
      settings: block_version=12.1
  DE1 : Subsystem
      mask Display: disp('z^{-1}','texmode','on')
  DE10 : Subsystem
      mask Display: disp('z^{-1}','texmode','on')
  DE11 : Subsystem
      mask Display: disp('z^{-1}','texmode','on')
  DE12 : Subsystem
      mask Display: disp('z^{-1}','texmode','on')
  DE13 : Subsystem
      mask Display: disp('z^{-1}','texmode','on')
  DE14 : Subsystem
      mask Display: disp('z^{-1}','texmode','on')
  DE15 : Subsystem
      mask Display: disp('z^{-1}','texmode','on')
  DE16 : Subsystem
      mask Display: disp('z^{-1}','texmode','on')
  DE17 : Subsystem
      mask Display: disp('z^{-1}','texmode','on')
  DE18 : Subsystem
      mask Display: disp('z^{-1}','texmode','on')
  DE19 : Subsystem
      mask Display: disp('z^{-1}','texmode','on')
  DE2 : Subsystem
      mask Display: disp('z^{-1}','texmode','on')
  DE20 : Subsystem
      mask Display: disp('z^{-1}','texmode','on')
  DE21 : Subsystem
      mask Display: disp('z^{-1}','texmode','on')
  DE22 : Subsystem
      mask Display: disp('z^{-1}','texmode','on')
  DE23 : Subsystem
      mask Display: disp('z^{-1}','texmode','on')
  DE24 : Subsystem
      mask Display: disp('z^{-1}','texmode','on')
  DE25 : Subsystem
      mask Display: disp('z^{-1}','texmode','on')
  DE26 : Subsystem
      mask Display: disp('z^{-1}','texmode','on')
  DE27 : Subsystem
      mask Display: disp('z^{-1}','texmode','on')
  DE28 : Subsystem
      mask Display: disp('z^{-1}','texmode','on')
  DE29 : Subsystem
      mask Display: disp('z^{-1}','texmode','on')
  DE3 : Subsystem
      mask Display: disp('z^{-1}','texmode','on')
  DE30 : Subsystem
      mask Display: disp('z^{-1}','texmode','on')
  DE4 : Subsystem
      mask Display: disp('z^{-1}','texmode','on')
  DE5 : Subsystem
      mask Display: disp('z^{-1}','texmode','on')
  DE6 : Subsystem
      mask Display: disp('z^{-1}','texmode','on')
  DE7 : Subsystem
      mask Display: disp('z^{-1}','texmode','on')
  DE8 : Subsystem
      mask Display: disp('z^{-1}','texmode','on')
  DE9 : Subsystem
      mask Display: disp('z^{-1}','texmode','on')
  Terminator : Terminator
  Out2 : Outport
  wires:
  Concat/1 -> Out2/1
  In1/1 -> 1to2/1(In)
  1to2/1(Out1) -> DE1/1(In1)
  DE30/1(Out1) -> Terminator/1
  1to2/2(Out2) -> Concat/31
  DE1/2(Out2) -> Concat/30
  DE2/2(Out2) -> Concat/29
  DE3/2(Out2) -> Concat/28
  DE4/2(Out2) -> Concat/27
  DE5/2(Out2) -> Concat/26
  DE6/2(Out2) -> Concat/25
  DE7/2(Out2) -> Concat/24
  DE8/2(Out2) -> Concat/23
  DE9/2(Out2) -> Concat/22
  DE10/2(Out2) -> Concat/21
  DE11/2(Out2) -> Concat/20
  DE12/2(Out2) -> Concat/19
  DE13/2(Out2) -> Concat/18
  DE14/2(Out2) -> Concat/17
  DE15/2(Out2) -> Concat/16
  DE16/2(Out2) -> Concat/15
  DE17/2(Out2) -> Concat/14
  DE18/2(Out2) -> Concat/13
  DE19/2(Out2) -> Concat/12
  DE20/2(Out2) -> Concat/11
  DE21/2(Out2) -> Concat/10
  DE22/2(Out2) -> Concat/9
  DE23/2(Out2) -> Concat/8
  DE24/2(Out2) -> Concat/7
  DE25/2(Out2) -> Concat/6
  DE26/2(Out2) -> Concat/5
  DE27/2(Out2) -> Concat/4
  DE28/2(Out2) -> Concat/3
  DE29/2(Out2) -> Concat/2
  DE30/2(Out2) -> Concat/1
  DE2/1(Out1) -> DE3/1(In1)
  DE3/1(Out1) -> DE4/1(In1)
  DE4/1(Out1) -> DE5/1(In1)
  DE5/1(Out1) -> DE6/1(In1)
  DE6/1(Out1) -> DE7/1(In1)
  DE7/1(Out1) -> DE8/1(In1)
  DE8/1(Out1) -> DE9/1(In1)
  DE9/1(Out1) -> DE10/1(In1)
  DE10/1(Out1) -> DE11/1(In1)
  DE11/1(Out1) -> DE12/1(In1)
  DE12/1(Out1) -> DE13/1(In1)
  DE13/1(Out1) -> DE14/1(In1)
  DE14/1(Out1) -> DE15/1(In1)
  DE15/1(Out1) -> DE16/1(In1)
  DE16/1(Out1) -> DE17/1(In1)
  DE17/1(Out1) -> DE18/1(In1)
  DE18/1(Out1) -> DE19/1(In1)
  DE19/1(Out1) -> DE20/1(In1)
  DE20/1(Out1) -> DE21/1(In1)
  DE21/1(Out1) -> DE22/1(In1)
  DE22/1(Out1) -> DE23/1(In1)
  DE23/1(Out1) -> DE24/1(In1)
  DE24/1(Out1) -> DE25/1(In1)
  DE25/1(Out1) -> DE26/1(In1)
  DE26/1(Out1) -> DE27/1(In1)
  DE27/1(Out1) -> DE28/1(In1)
  DE28/1(Out1) -> DE29/1(In1)
  DE29/1(Out1) -> DE30/1(In1)
  DE1/1(Out1) -> DE2/1(In1)

== system receiver_overall_reset/Receiver/Sym-Chooser/1-9/Corr0/Corr ==
  In1 : Inport
  AddSub{,1..6} (7 alike) : xbsIndex_r4/AddSub  mode=Addition  use_carryin=off  use_carryout=off  en=off  latency=0  precision=Full  arith_type=Unsigned  n_bits=16  bin_pt=14  quantization=Truncate  overflow=Wrap  dbl_ovrd=off  use_behavioral_HDL=off  hw_selection=Fabric  pipelined=off  block_type=addsub
      AddSub settings: xl_area=[2 0 0 3 0 0 0]  block_version=12.1
      AddSub1 settings: xl_area=[2 0 0 3 0 0 0]  block_version=12.1
      AddSub2 settings: xl_area=[3 0 0 4 0 0 0]  block_version=12.1
      AddSub3 settings: xl_area=[3 0 0 5 0 0 0]  block_version=12.1
      AddSub4 settings: xl_area=[2 0 0 3 0 0 0]  block_version=12.1
      AddSub5 settings: xl_area=[2 0 0 3 0 0 0]  block_version=12.1
      AddSub6 settings: xl_area=[3 0 0 4 0 0 0]  block_version=12.1
  LUT{0..7} (8 alike) : xbsIndex_r4/ROM  depth=16  initVector=[0,1,1,2,1,2,2,3,1,2,2,3,2,3,3,4]  distributed_mem=Distributed memory  rst=off  init_reg=0  en=off  latency=0  arith_type=Unsigned  n_bits=3  bin_pt=0  dbl_ovrd=off  optimize=Area  use_rpm=on  block_type=sprom
      settings: xl_area=[0 0 1 0 0 0 0]  block_version=12.1
  Slice0 : xbsIndex_r4/Slice  nbits=4  boolean_output=off  mode=Lower Bit Location + Width  bit1=0  base1=MSB of Input  bit0=0  base0=LSB of Input  dbl_ovrd=off  block_type=slice
      settings: block_version=12.1
  Slice1 : xbsIndex_r4/Slice  nbits=4  boolean_output=off  mode=Lower Bit Location + Width  bit1=-4  base1=MSB of Input  bit0=4  base0=LSB of Input  dbl_ovrd=off  block_type=slice
      settings: block_version=12.1
  Slice2 : xbsIndex_r4/Slice  nbits=4  boolean_output=off  mode=Lower Bit Location + Width  bit1=-8  base1=MSB of Input  bit0=8  base0=LSB of Input  dbl_ovrd=off  block_type=slice
      settings: block_version=12.1
  Slice3 : xbsIndex_r4/Slice  nbits=4  boolean_output=off  mode=Lower Bit Location + Width  bit1=-12  base1=MSB of Input  bit0=12  base0=LSB of Input  dbl_ovrd=off  block_type=slice
      settings: block_version=12.1
  Slice4 : xbsIndex_r4/Slice  nbits=4  boolean_output=off  mode=Lower Bit Location + Width  bit1=0  base1=LSB of Input  bit0=16  base0=LSB of Input  dbl_ovrd=off  block_type=slice
      settings: block_version=12.1
  Slice5 : xbsIndex_r4/Slice  nbits=4  boolean_output=off  mode=Lower Bit Location + Width  bit1=0  base1=LSB of Input  bit0=20  base0=LSB of Input  dbl_ovrd=off  block_type=slice
      settings: block_version=12.1
  Slice6 : xbsIndex_r4/Slice  nbits=4  boolean_output=off  mode=Lower Bit Location + Width  bit1=0  base1=LSB of Input  bit0=24  base0=LSB of Input  dbl_ovrd=off  block_type=slice
      settings: block_version=12.1
  Slice7 : xbsIndex_r4/Slice  nbits=4  boolean_output=off  mode=Lower Bit Location + Width  bit1=0  base1=LSB of Input  bit0=28  base0=LSB of Input  dbl_ovrd=off  block_type=slice
      settings: block_version=12.1
  Out2 : Outport
  wires:
  In1/1 -> Slice0/1, Slice1/1, Slice2/1, Slice7/1, Slice6/1, Slice3/1, Slice4/1, Slice5/1
  Slice0/1 -> LUT0/1
  Slice3/1 -> LUT3/1
  Slice2/1 -> LUT2/1
  Slice1/1 -> LUT1/1
  LUT0/1 -> AddSub/1
  LUT1/1 -> AddSub/2
  LUT2/1 -> AddSub1/1
  LUT3/1 -> AddSub1/2
  AddSub1/1 -> AddSub2/2
  AddSub/1 -> AddSub2/1
  AddSub3/1 -> Out2/1
  Slice4/1 -> LUT4/1
  Slice7/1 -> LUT7/1
  Slice6/1 -> LUT6/1
  Slice5/1 -> LUT5/1
  LUT4/1 -> AddSub4/1
  LUT5/1 -> AddSub4/2
  LUT6/1 -> AddSub5/1
  LUT7/1 -> AddSub5/2
  AddSub5/1 -> AddSub6/2
  AddSub4/1 -> AddSub6/1
  AddSub2/1 -> AddSub3/1
  AddSub6/1 -> AddSub3/2

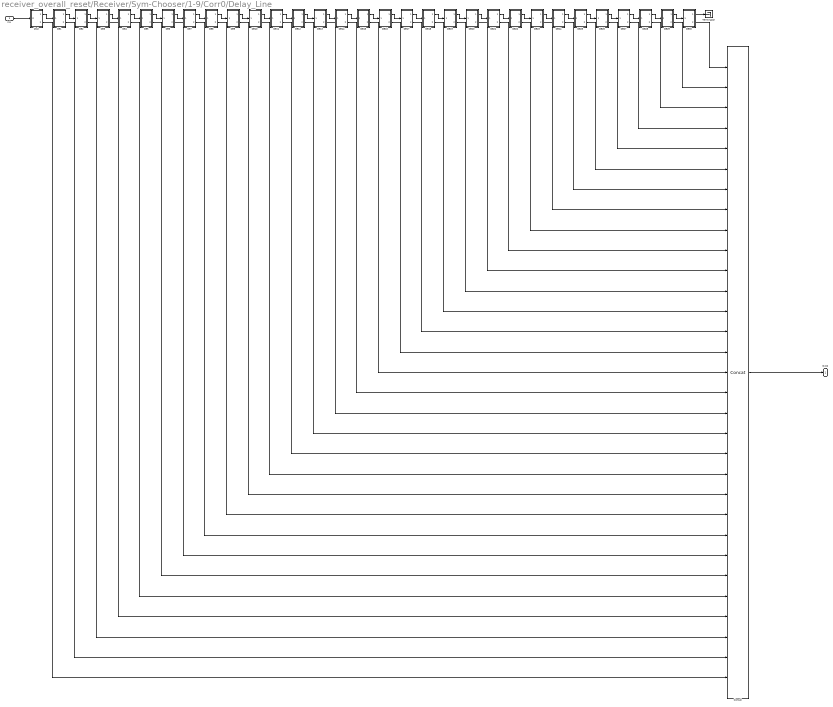
== system receiver_overall_reset/Receiver/Sym-Chooser/1-9/Corr0/Delay_Line ==
  In1 : Inport
  1to2 : Subsystem
  Concat : xbsIndex_r4/Concat  num_inputs=31  dbl_ovrd=off  block_type=concat
      settings: block_version=12.1
  DE1 : Subsystem
      mask Display: disp('z^{-1}','texmode','on')
  DE10 : Subsystem
      mask Display: disp('z^{-1}','texmode','on')
  DE11 : Subsystem
      mask Display: disp('z^{-1}','texmode','on')
  DE12 : Subsystem
      mask Display: disp('z^{-1}','texmode','on')
  DE13 : Subsystem
      mask Display: disp('z^{-1}','texmode','on')
  DE14 : Subsystem
      mask Display: disp('z^{-1}','texmode','on')
  DE15 : Subsystem
      mask Display: disp('z^{-1}','texmode','on')
  DE16 : Subsystem
      mask Display: disp('z^{-1}','texmode','on')
  DE17 : Subsystem
      mask Display: disp('z^{-1}','texmode','on')
  DE18 : Subsystem
      mask Display: disp('z^{-1}','texmode','on')
  DE19 : Subsystem
      mask Display: disp('z^{-1}','texmode','on')
  DE2 : Subsystem
      mask Display: disp('z^{-1}','texmode','on')
  DE20 : Subsystem
      mask Display: disp('z^{-1}','texmode','on')
  DE21 : Subsystem
      mask Display: disp('z^{-1}','texmode','on')
  DE22 : Subsystem
      mask Display: disp('z^{-1}','texmode','on')
  DE23 : Subsystem
      mask Display: disp('z^{-1}','texmode','on')
  DE24 : Subsystem
      mask Display: disp('z^{-1}','texmode','on')
  DE25 : Subsystem
      mask Display: disp('z^{-1}','texmode','on')
  DE26 : Subsystem
      mask Display: disp('z^{-1}','texmode','on')
  DE27 : Subsystem
      mask Display: disp('z^{-1}','texmode','on')
  DE28 : Subsystem
      mask Display: disp('z^{-1}','texmode','on')
  DE29 : Subsystem
      mask Display: disp('z^{-1}','texmode','on')
  DE3 : Subsystem
      mask Display: disp('z^{-1}','texmode','on')
  DE30 : Subsystem
      mask Display: disp('z^{-1}','texmode','on')
  DE4 : Subsystem
      mask Display: disp('z^{-1}','texmode','on')
  DE5 : Subsystem
      mask Display: disp('z^{-1}','texmode','on')
  DE6 : Subsystem
      mask Display: disp('z^{-1}','texmode','on')
  DE7 : Subsystem
      mask Display: disp('z^{-1}','texmode','on')
  DE8 : Subsystem
      mask Display: disp('z^{-1}','texmode','on')
  DE9 : Subsystem
      mask Display: disp('z^{-1}','texmode','on')
  Terminator : Terminator
  Out2 : Outport
  wires:
  Concat/1 -> Out2/1
  In1/1 -> 1to2/1(In)
  1to2/1(Out1) -> DE1/1(In1)
  DE30/1(Out1) -> Terminator/1
  1to2/2(Out2) -> Concat/31
  DE1/2(Out2) -> Concat/30
  DE2/2(Out2) -> Concat/29
  DE3/2(Out2) -> Concat/28
  DE4/2(Out2) -> Concat/27
  DE5/2(Out2) -> Concat/26
  DE6/2(Out2) -> Concat/25
  DE7/2(Out2) -> Concat/24
  DE8/2(Out2) -> Concat/23
  DE9/2(Out2) -> Concat/22
  DE10/2(Out2) -> Concat/21
  DE11/2(Out2) -> Concat/20
  DE12/2(Out2) -> Concat/19
  DE13/2(Out2) -> Concat/18
  DE14/2(Out2) -> Concat/17
  DE15/2(Out2) -> Concat/16
  DE16/2(Out2) -> Concat/15
  DE17/2(Out2) -> Concat/14
  DE18/2(Out2) -> Concat/13
  DE19/2(Out2) -> Concat/12
  DE20/2(Out2) -> Concat/11
  DE21/2(Out2) -> Concat/10
  DE22/2(Out2) -> Concat/9
  DE23/2(Out2) -> Concat/8
  DE24/2(Out2) -> Concat/7
  DE25/2(Out2) -> Concat/6
  DE26/2(Out2) -> Concat/5
  DE27/2(Out2) -> Concat/4
  DE28/2(Out2) -> Concat/3
  DE29/2(Out2) -> Concat/2
  DE30/2(Out2) -> Concat/1
  DE2/1(Out1) -> DE3/1(In1)
  DE3/1(Out1) -> DE4/1(In1)
  DE4/1(Out1) -> DE5/1(In1)
  DE5/1(Out1) -> DE6/1(In1)
  DE6/1(Out1) -> DE7/1(In1)
  DE7/1(Out1) -> DE8/1(In1)
  DE8/1(Out1) -> DE9/1(In1)
  DE9/1(Out1) -> DE10/1(In1)
  DE10/1(Out1) -> DE11/1(In1)
  DE11/1(Out1) -> DE12/1(In1)
  DE12/1(Out1) -> DE13/1(In1)
  DE13/1(Out1) -> DE14/1(In1)
  DE14/1(Out1) -> DE15/1(In1)
  DE15/1(Out1) -> DE16/1(In1)
  DE16/1(Out1) -> DE17/1(In1)
  DE17/1(Out1) -> DE18/1(In1)
  DE18/1(Out1) -> DE19/1(In1)
  DE19/1(Out1) -> DE20/1(In1)
  DE20/1(Out1) -> DE21/1(In1)
  DE21/1(Out1) -> DE22/1(In1)
  DE22/1(Out1) -> DE23/1(In1)
  DE23/1(Out1) -> DE24/1(In1)
  DE24/1(Out1) -> DE25/1(In1)
  DE25/1(Out1) -> DE26/1(In1)
  DE26/1(Out1) -> DE27/1(In1)
  DE27/1(Out1) -> DE28/1(In1)
  DE28/1(Out1) -> DE29/1(In1)
  DE29/1(Out1) -> DE30/1(In1)
  DE1/1(Out1) -> DE2/1(In1)
